simulink model "trans_123_alphabeta_dq_V1"  (R2022a)
settings: Solver=FixedStepDiscrete  StartTime=0.0  StopTime=0.2  RelTol=1e-3
InitFcn:
  | Ts_xadc = 0.1;
values from neighbouring files (symbols this model uses):
  T_50MHz = 1/f_50MHz    (= 2e-08)    [trans_123_alphabeta_dq_params.m]
libraries: simulink x4
settings Model: DataTypeOverride=Off  Creator=trichte  LastModifiedBy=Andre Merx
settings SolverCC: AlgebraicLoopSolver=TrustRegion
settings DataIOCC: LimitDataPoints=on  SaveFormat=Array  SaveOutput=off  SaveTime=off  ReturnWorkspaceOutputs=off
settings OptimizationCC: BlockReduction=off  ConditionallyExecuteInputs=off  DefaultParameterBehavior=Inlined  LifeSpan=inf
settings DebuggingCC: AlgebraicLoopMsg=error  SolverPrmCheckMsg=warning  SingleTaskRateTransMsg=error  UnconnectedInputMsg=warning  UnconnectedOutputMsg=warning  UnconnectedLineMsg=warning  AllowSymbolicDim=off  StrictBusMsg=ErrorOnBusTreatedAsVector  SFUnexpectedBacktrackingDiag=warning  SFNoUnconditionalDefaultTransitionDiag=warning  SFExecutionAtInitializationDiag=none  SFMachineParentedDataDiag=warning  ArithmeticOperatorsInVariantConditions=warning
settings HardwareCC: ProdBitPerPointer=32  ProdBitPerSizeT=32  ProdBitPerPtrDiffT=32  ProdLargestAtomicFloat=None  ProdIntDivRoundTo=Undefined  ProdEndianess=Unspecified  ProdWordSize=32  ProdHWDeviceType=ASIC/FPGA->ASIC/FPGA  ProdEqTarget=off
settings ModelReferenceCC: PropagateSignalLabelsOutOfModel=off
settings SFSimCC: SimUseLocalCustomCode=off  CustomCodeUndefinedFunction=UseInterfaceOnly
settings RTWCC: RTWUseLocalCustomCode=off
settings CodeAppCC: StateflowObjectComments=on
settings GRTTargetCC: TargetLangStandard=C89/C90 (ANSI)
settings ConfigComp: CovMetricSettings=dw  CovSaveCumulativeToWorkspaceVar=on  CovSaveSingleToWorkspaceVar=on  CovExternalEMLEnable=off  CovSFcnEnable=off

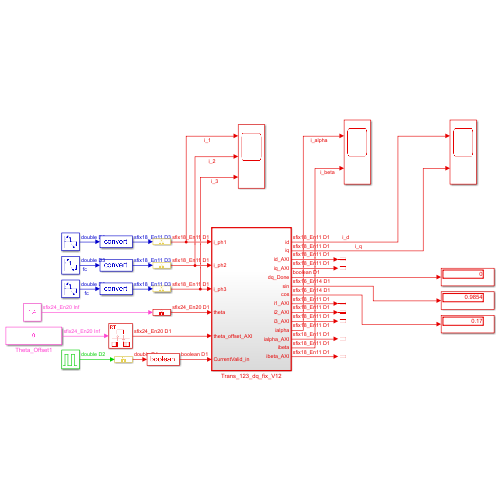
[thumbnail: Simulink's stored preview of the top-level diagram]
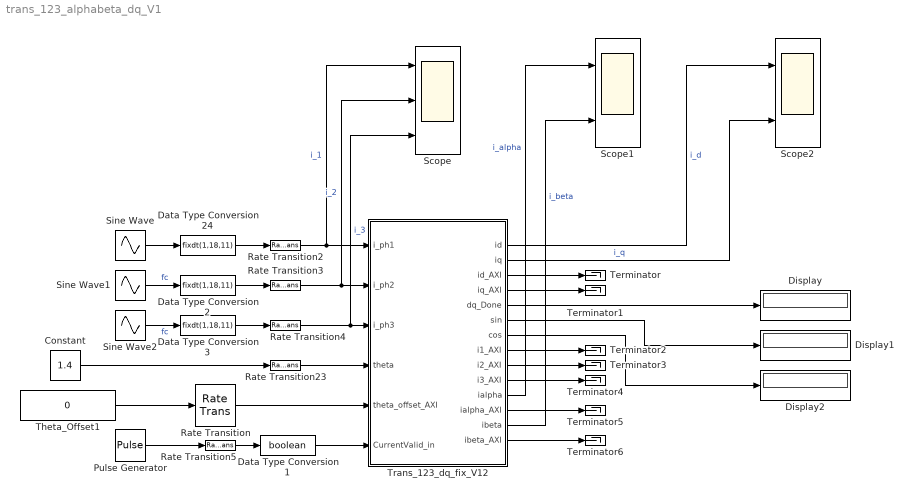
== system trans_123_alphabeta_dq_V1 ==
  Constant : Constant  Value=1.4  OutDataTypeStr=fixdt(1,24,20)
  Data Type Conversion1 : DataTypeConversion  OutDataTypeStr=boolean  SaturateOnIntegerOverflow=off  RndMeth=Floor
  Data Type Conversion2 : DataTypeConversion  OutDataTypeStr=fixdt(1,18,11)  SaturateOnIntegerOverflow=off  RndMeth=Floor
  Data Type Conversion24 : DataTypeConversion  OutDataTypeStr=fixdt(1,18,11)  SaturateOnIntegerOverflow=off  RndMeth=Floor
  Data Type Conversion3 : DataTypeConversion  OutDataTypeStr=fixdt(1,18,11)  SaturateOnIntegerOverflow=off  RndMeth=Floor
  Display : Display
  Display1 : Display
  Display2 : Display
  Pulse Generator : DiscretePulseGenerator  PulseType=Time based  Period=1/100000  PulseWidth=5
  Rate Transition{,2..5,23} (6 alike) : RateTransition  OutPortSampleTime=T_50MHz
  Scope : Scope  NumInputPorts=3
  Scope1 : Scope  NumInputPorts=2
  Scope2 : Scope  NumInputPorts=2
  Sine Wave : Sin  Frequency=100  SampleTime=1/100000
  Sine Wave1 : Sin  Frequency=100  Phase=(2/3)*pi  SampleTime=1/100000
  Sine Wave2 : Sin  Frequency=100  Phase=(4/3)*pi  SampleTime=1/100000
  Terminator{,1..6} (7 alike) : Terminator
  Theta_Offset1 : Constant  Value=0  OutDataTypeStr=fixdt(1,24,20)
  Trans_123_dq_fix_V12 : Subsystem  TreatAsAtomicUnit=on
  wires:
  Sine Wave2/1 -> Data Type Conversion3/1  "fc"
  Trans_123_dq_fix_V12/13(ibeta) -> Scope1/2  "i_beta"
  Trans_123_dq_fix_V12/3(id_AXI) -> Terminator/1
  Trans_123_dq_fix_V12/5(dq_Done) -> Display/1
  Trans_123_dq_fix_V12/8(i1_AXI) -> Terminator2/1
  Trans_123_dq_fix_V12/1(id) -> Scope2/1  "i_d"
  Theta_Offset1/1 -> Rate Transition/1
  Rate Transition3/1 -> Scope/2, Trans_123_dq_fix_V12/2(i_ph2)  "i_2"
  Rate Transition2/1 -> Scope/1, Trans_123_dq_fix_V12/1(i_ph1)  "i_1"
  Rate Transition/1 -> Trans_123_dq_fix_V12/5(theta_offset_AXI)
  Data Type Conversion1/1 -> Trans_123_dq_fix_V12/6(CurrentValid_in)
  Rate Transition4/1 -> Scope/3, Trans_123_dq_fix_V12/3(i_ph3)  "i_3"
  Pulse Generator/1 -> Rate Transition5/1
  Trans_123_dq_fix_V12/9(i2_AXI) -> Terminator3/1
  Rate Transition23/1 -> Trans_123_dq_fix_V12/4(theta)
  Trans_123_dq_fix_V12/4(iq_AXI) -> Terminator1/1
  Trans_123_dq_fix_V12/7(cos) -> Display2/1
  Constant/1 -> Rate Transition23/1
  Trans_123_dq_fix_V12/14(ibeta_AXI) -> Terminator6/1
  Trans_123_dq_fix_V12/11(ialpha) -> Scope1/1  "i_alpha"
  Trans_123_dq_fix_V12/10(i3_AXI) -> Terminator4/1
  Rate Transition5/1 -> Data Type Conversion1/1
  Trans_123_dq_fix_V12/2(iq) -> Scope2/2  "i_q"
  Trans_123_dq_fix_V12/6(sin) -> Display1/1
  Trans_123_dq_fix_V12/12(ialpha_AXI) -> Terminator5/1
  Sine Wave/1 -> Data Type Conversion24/1
  Data Type Conversion24/1 -> Rate Transition2/1
  Data Type Conversion2/1 -> Rate Transition3/1
  Data Type Conversion3/1 -> Rate Transition4/1
  Sine Wave1/1 -> Data Type Conversion2/1  "fc"

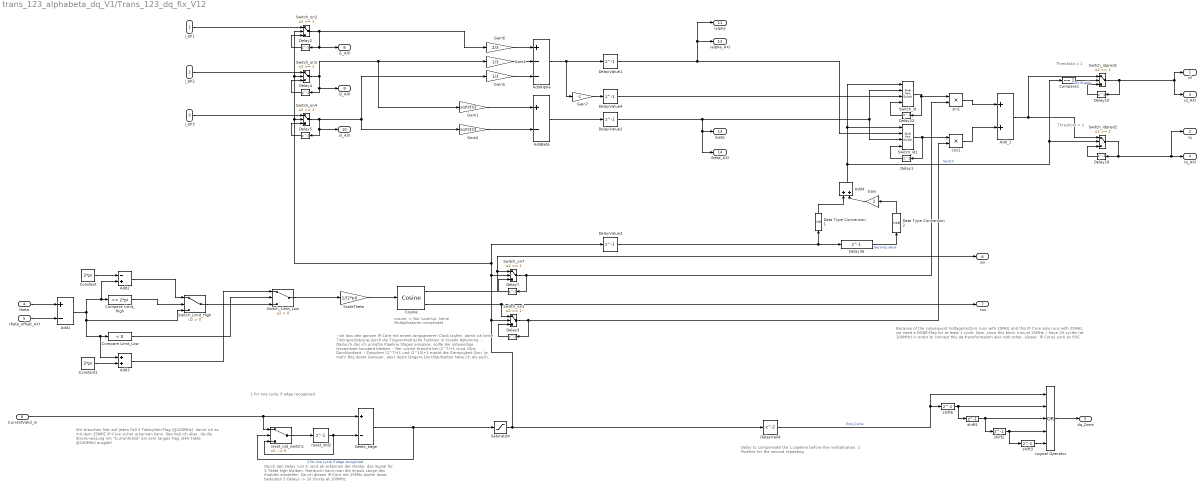
== system trans_123_alphabeta_dq_V1/Trans_123_dq_fix_V12 ==
  note: Delay to compensate the 1 pipeline before the multiplication.
      | 1 Pipeline for the second repeating.
  note: cosine -> Nur Look-Up,
      | keine Multiplikatoren
      | verwendet
  note: - Ich lass den ganzen IP Core mit einem langsameren Clock laufen,
      | damit ich keine Timingverletzung durch die Trigonometrische
      | Funktion in Vivado bekomme.
      | - Dadurch das ich unnütze Pipeline Stages einspare, sollte
      | die notwendige Gesamtzeit konstant bleiben.
      | - Der cosine braucht bei (2^7)+1 circa 24ns Durchlaufzeit.
      | - Zwischen (2^7)+1 und (2^13)+1 macht die Genauigkeit Sinn. Je mehr Bits
      | desto Genauer, aber desto längere Durchlaufzeiten habe ich als auch mehr
      | Ressourcen brauche ich. (Habe mich aktuell für (2^9)+1 entschieden.
  note: Durch den Delay von 5, wird ab erkennen der Flanke,
      |  das Signal für 5 Takte high bleiben.
      | Hierdurch kann man die Impuls Länge des Enables einstellen.
      | Da ich diesen IP-Core mit 25MHz laufen lasse, bedeuten 5 Delays -> 20 Clocks at 100MHz
  note: 1 for one cycle if edge recognized
  note: Wir brauchen hier auf jeden Fall 4 Taktzyklen-Flag (@100MHz),
      | damit ich es mit dem 25MHZ IP-Core sicher erkennen kann. Das hab
      | ich aber, da die Strommessung mit "CurrentValid" ein sehr langes Flag
      | (345 Takte @100MHz) ausgibt!
  note: Because of the subsequent VoltageVectors runs with 25MHz and this
      | IP Core also runs with 25MHz, we need a DONE-Flag for at least 1 cycle.
      | Now, since this block runs at 25MHz, i have 20 cycles (at 100MHz) in order
      | to connect this dq-transformation also with other, slower, IP Cores such as
      | FOC.
  note: Threshold = 1
  note: Threshold = 2
  i_ph1 : Inport
  i_ph2 : Inport  Port=2
  i_ph3 : Inport  Port=3
  theta : Inport  Port=4
  theta_offset_AXI : Inport  Port=5
  CurrentValid_in : Inport  Port=6
  Add1 : Sum  Inputs=+-  OutDataTypeStr=Inherit: Same as accumulator
  Add2 : Sum  Inputs=-+  OutDataTypeStr=Inherit: Same as first input
  Add3 : Sum  OutDataTypeStr=Inherit: Same as first input
  Add4 : Sum  AccumDataTypeStr=int8  OutDataTypeStr=int8  RndMeth=Simplest
  AddAlpha : Sum  Inputs=+--  OutDataTypeStr=Inherit: Same as accumulator
  AddBeta : Sum  Inputs=+-  OutDataTypeStr=Inherit: Same as accumulator
  Add_1 : Sum  OutDataTypeStr=Inherit: Same as accumulator
  Compare Limit_High : simulink/Logic and Bit Operations/Compare To Constant  relop=>=  const=2*pi  OutDataTypeStr=boolean
  Compare Limit_Low : simulink/Logic and Bit Operations/Compare To Constant  relop=<  const=0  OutDataTypeStr=boolean
  Compare1 : simulink/Logic and Bit Operations/Compare To Constant  relop===  const=1  OutDataTypeStr=boolean
  Constant : Constant  Value=2*pi  OutDataTypeStr=fixdt(1,24,20)  SampleTime=T_50MHz
  Constant1 : Constant  Value=2*pi  OutDataTypeStr=fixdt(1,24,20)  SampleTime=T_50MHz
  Cosine : simulink/Lookup Tables/Cosine  Formula=sin(2*pi*u) and cos(2*pi*u)  NumDataPoints=(2^9)+1  OutputWordLength=16  InternalRulePriority=Precision
      settings: SourceProductBaseCode=SL
  Data Type Conversion1 : DataTypeConversion  OutDataTypeStr=int8  SaturateOnIntegerOverflow=off  RndMeth=Floor
  Data Type Conversion2 : DataTypeConversion  OutDataTypeStr=int8  SaturateOnIntegerOverflow=off  RndMeth=Floor
  Delay{1..5,7,10,16,22,36} (10 alike) : Delay  DelayLength=1
  DelayValid : Delay
  DelayValue{1..4} (4 alike) : Delay  DelayLength=1
  Detec_edge : Sum  Inputs=+-  AccumDataTypeStr=int8  OutDataTypeStr=int8
  Gain : Gain  Gain=2  RndMeth=Simplest
  Gain1 : Gain  Gain=sqrt(3)/3  OutDataTypeStr=Inherit: Same as input
  Gain2 : Gain  Gain=sqrt(3)/3  OutDataTypeStr=Inherit: Same as input
  Gain4 : Gain  Gain=1/3  OutDataTypeStr=Inherit: Same as input
  Gain5 : Gain  Gain=1/3  OutDataTypeStr=Inherit: Same as input
  Gain6 : Gain  Gain=2/3  OutDataTypeStr=Inherit: Same as input
  Gain7 : Gain  Gain=-1  OutDataTypeStr=Inherit: Same as input
  Logical Operator : Logic  Operator=OR  Inputs=5  AllPortsSameDT=off  OutDataTypeStr=boolean
  Saturation : Saturate  UpperLimit=1  LowerLimit=0  OutMin=[0]  OutMax=[1]  OutDataTypeStr=fixdt(0,1)
  ScaleTheta : Gain  Gain=1/(2*pi)  OutDataTypeStr=Inherit: Same as input
  Switch_Limit_High : Switch  Criteria=u2 > Threshold  OutDataTypeStr=fixdt(1,24,20)  SaturateOnIntegerOverflow=off  InputSameDT=off
  Switch_Limit_Low : Switch  Criteria=u2 > Threshold  OutDataTypeStr=fixdt(1,24,20)  SaturateOnIntegerOverflow=off  InputSameDT=off
  Switch_id : MultiPortSwitch  Inputs=2  DataPortForDefault=Additional data port  DiagnosticForDefault=None  OutDataTypeStr=Inherit: Inherit via back propagation  RndMeth=Simplest  SaturateOnIntegerOverflow=off  InputSameDT=off
  Switch_id1 : MultiPortSwitch  Inputs=2  DataPortForDefault=Additional data port  DiagnosticForDefault=None  OutDataTypeStr=Inherit: Inherit via back propagation  RndMeth=Simplest  SaturateOnIntegerOverflow=off  InputSameDT=off
  Switch_idpred1 : Switch  Threshold=1  OutDataTypeStr=Inherit: Inherit via back propagation  RndMeth=Simplest  SaturateOnIntegerOverflow=off  InputSameDT=off
  Switch_idpred2 : Switch  Threshold=2  OutDataTypeStr=Inherit: Inherit via back propagation  RndMeth=Simplest  SaturateOnIntegerOverflow=off  InputSameDT=off
  Switch_on1 : Switch  Threshold=1  OutDataTypeStr=fixdt(1,16,14)  SaturateOnIntegerOverflow=off  InputSameDT=off
  Switch_on2 : Switch  Threshold=1  OutDataTypeStr=Inherit: Inherit via back propagation  RndMeth=Simplest  SaturateOnIntegerOverflow=off  InputSameDT=off
  Switch_on3 : Switch  Threshold=1  OutDataTypeStr=Inherit: Inherit via back propagation  RndMeth=Simplest  SaturateOnIntegerOverflow=off  InputSameDT=off
  Switch_on4 : Switch  Threshold=1  OutDataTypeStr=Inherit: Inherit via back propagation  RndMeth=Simplest  SaturateOnIntegerOverflow=off  InputSameDT=off
  Switch_on7 : Switch  Threshold=1  OutDataTypeStr=fixdt(1,16,14)  SaturateOnIntegerOverflow=off  InputSameDT=off
  cos1 : Product  RndMeth=Simplest  OutDataTypeStr=Inherit: Same as first input
  reset_old2 : Delay  DelayLength=1
  reset_old_switch1 : Switch  Criteria=u2 ~= 0  SaturateOnIntegerOverflow=off  InputSameDT=off
  shift{1..3,6} (4 alike) : Delay  DelayLength=1
  sin1 : Product  RndMeth=Simplest  OutDataTypeStr=Inherit: Same as first input
  id : Outport  VectorParamsAs1DForOutWhenUnconnected=off
  iq : Outport  Port=2  VectorParamsAs1DForOutWhenUnconnected=off
  id_AXI : Outport  Port=3  VectorParamsAs1DForOutWhenUnconnected=off
  iq_AXI : Outport  Port=4  VectorParamsAs1DForOutWhenUnconnected=off
  dq_Done : Outport  Port=5  VectorParamsAs1DForOutWhenUnconnected=off
  sin : Outport  Port=6  VectorParamsAs1DForOutWhenUnconnected=off
  cos : Outport  Port=7  VectorParamsAs1DForOutWhenUnconnected=off
  i1_AXI : Outport  Port=8  VectorParamsAs1DForOutWhenUnconnected=off
  i2_AXI : Outport  Port=9  VectorParamsAs1DForOutWhenUnconnected=off
  i3_AXI : Outport  Port=10  VectorParamsAs1DForOutWhenUnconnected=off
  ialpha : Outport  Port=11  VectorParamsAs1DForOutWhenUnconnected=off
  ialpha_AXI : Outport  Port=12  VectorParamsAs1DForOutWhenUnconnected=off
  ibeta : Outport  Port=13  VectorParamsAs1DForOutWhenUnconnected=off
  ibeta_AXI : Outport  Port=14  VectorParamsAs1DForOutWhenUnconnected=off
  wires:
  Gain1/1 -> AddBeta/1
  Gain2/1 -> AddBeta/2
  theta/1 -> Add1/1
  Add1/1 -> Switch_Limit_High/3, Add3/1, Compare Limit_Low/1, Add2/2, Compare Limit_High/1
  theta_offset_AXI/1 -> Add1/2
  Switch_Limit_High/1 -> Switch_Limit_Low/3
  Compare Limit_High/1 -> Switch_Limit_High/2
  Compare Limit_Low/1 -> Switch_Limit_Low/2
  Constant/1 -> Add2/1
  Add2/1 -> Switch_Limit_High/1
  Constant1/1 -> Add3/2
  Add3/1 -> Switch_Limit_Low/1
  Switch_idpred2/1 -> iq/1, iq_AXI/1, Delay16/1
  Switch_idpred1/1 -> Delay10/1, id/1, id_AXI/1
  Saturation/1 -> DelayValid/1, Switch_on1/2, Switch_on7/2, DelayValue3/1, Switch_on2/2, Switch_on3/2, Switch_on4/2
  Delay3/1 -> Switch_on1/3
  Delay7/1 -> Switch_on7/3
  ScaleTheta/1 -> Cosine/1
  Cosine/2 -> cos/1, Switch_on1/1
  Switch_on7/1 -> Delay7/1, sin1/2
  Cosine/1 -> sin/1, Switch_on7/1
  Switch_on1/1 -> Delay3/1, cos1/2
  Switch_Limit_Low/1 -> ScaleTheta/1
  Gain4/1 -> AddAlpha/2
  Gain5/1 -> AddAlpha/3
  Gain6/1 -> AddAlpha/1
  Detec_edge/1 -> Saturation/1, reset_old_switch1/2  "1 for one cycle if edge recognized"
  reset_old2/1 -> reset_old_switch1/3, Detec_edge/2
  CurrentValid_in/1 -> reset_old_switch1/1, Detec_edge/1
  reset_old_switch1/1 -> reset_old2/1
  Delay2/1 -> Switch_on2/3
  Switch_on2/1 -> Delay2/1, i1_AXI/1, Gain6/1
  i_ph1/1 -> Switch_on2/1
  Switch_on3/1 -> i2_AXI/1, Delay4/1, Gain1/1, Gain4/1
  Delay4/1 -> Switch_on3/3
  i_ph2/1 -> Switch_on3/1
  Switch_on4/1 -> i3_AXI/1, Delay5/1, Gain2/1, Gain5/1
  Delay5/1 -> Switch_on4/3
  i_ph3/1 -> Switch_on4/1
  AddAlpha/1 -> Gain7/1, DelayValue1/1
  AddBeta/1 -> DelayValue2/1
  DelayValid/1 -> shift6/1, Logical Operator/1  "End_Cycle"
  shift6/1 -> Logical Operator/2, shift1/1
  Logical Operator/1 -> dq_Done/1
  Delay10/1 -> Switch_idpred1/3
  Delay16/1 -> Switch_idpred2/3
  Compare1/1 -> Switch_idpred1/2  "id1-Enable"
  Delay22/1 -> Switch_id/4
  Add4/1 -> Switch_idpred2/2, Compare1/1, Switch_id1/1, Switch_id/1  "Switch"
  sin1/1 -> Add_1/1
  cos1/1 -> Add_1/2
  DelayValue1/1 -> ialpha/1, ialpha_AXI/1, Switch_id1/2
  Switch_id/1 -> sin1/1, Delay22/1
  Delay1/1 -> Switch_id1/4
  Switch_id1/1 -> cos1/1, Delay1/1
  DelayValue3/1 -> Data Type Conversion1/1, Delay36/1
  Data Type Conversion1/1 -> Add4/1
  Gain/1 -> Add4/2
  Delay36/1 -> Data Type Conversion2/1  "Second_value"
  Data Type Conversion2/1 -> Gain/1
  DelayValue2/1 -> ibeta_AXI/1, ibeta/1, Switch_id/2, Switch_id1/3
  Add_1/1 -> Switch_idpred1/1, Switch_idpred2/1
  DelayValue4/1 -> Switch_id/3
  Gain7/1 -> DelayValue4/1
  shift1/1 -> Logical Operator/3, shift2/1
  shift2/1 -> shift3/1, Logical Operator/4
  shift3/1 -> Logical Operator/5
